simulink model "Modelo_asynchronous_machine_with_inverter"  (R2023b)
settings: Solver=ode45  StartTime=0.0  StopTime=0.5  MaxStep=1e-5  RelTol=1e-3
libraries: spsIGBTDiodeLib x6, spsVoltageMeasurementLib x3, spsAsynchronousMachineSIUnitsLib x1, simulink x1, spsDCVoltageSourceLib x1, spsThreePhaseVIMeasurementLib x1, spspowerguiLib x1
settings Model: Creator=HP  LastModifiedBy=HP

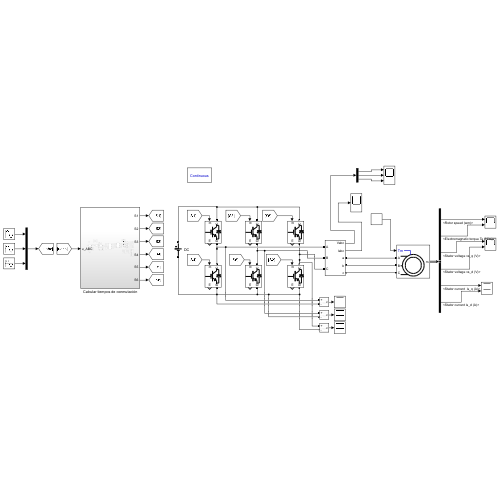
[thumbnail: Simulink's stored preview of the top-level diagram]
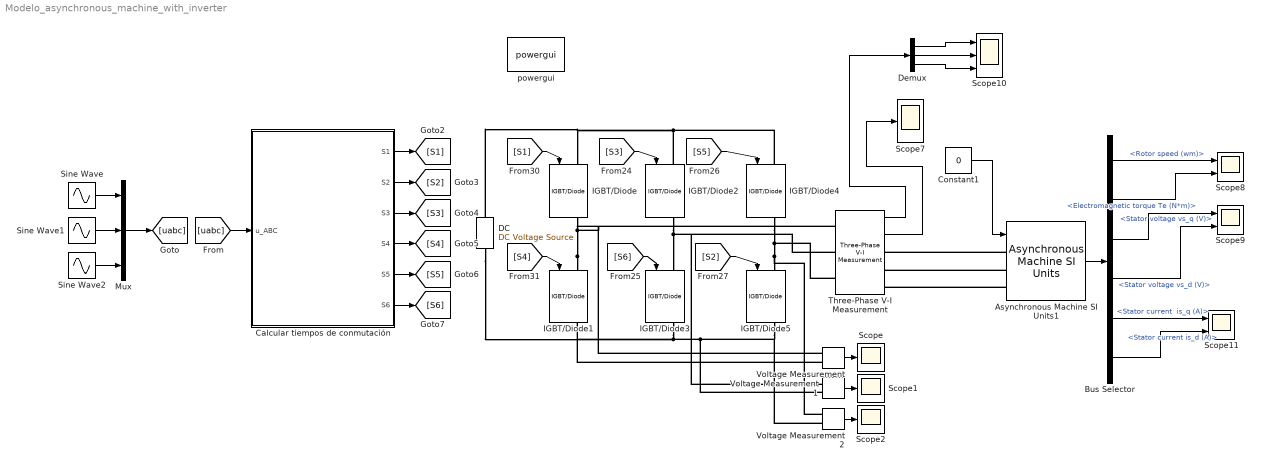
== system Modelo_asynchronous_machine_with_inverter ==
  Asynchronous Machine SI Units1 : spsAsynchronousMachineSIUnitsLib/Asynchronous Machine SI Units  RotorType=Squirrel-cage  PresetModel="01:  5 HP   460 V 60Hz 1750 RPM"  MechanicalLoad=Torque Tm  ShowDetailedParameters=on  ReferenceFrame=Rotor  Units=SI  MeasurementBus=off  NominalParameters=[3730 460 60]  VoltageRatio=1  Stator=[1.115 0.005974]  Rotor=[1.083 0.005974]  Cage1=[0.4155 0.002066]  Cage2=[0.4168 0.0003495]  Lm=0.2037  Mechanical=[0.02 0.005752 2]  PolePairs=2  InitialConditions=[1 0 0 0 0 0 0 0]  SimulateSaturation=off  Saturation=[14.03593122, 27.81365428, 53.79336849, 72.68890987, 97.98006896, 148.6815601, 215.7428561, 302.9841135, 428.7778367 ; 230, 322, 414, 460, 506, 552, 598, 644, 690]  LoadFlowParameters=1492000  TsPowergui=0  TsBlock=-1  IterativeModel=Trapezoidal non iterative  IterativeDiscreteModel=Trapezoidal non iterative  Pmec=1.492e+006
  Bus Selector : BusSelector  OutputSignals="Mechanical.Rotor speed (wm),Mechanical.Electromagnetic torque Te (N*m),Stator measurements.Stator voltage vs_q (V),Stator measurements.Stator voltage vs_d (V),Stator measurements.Stator current  is_q (A),Stator measurements.Stator current is_d (A)"
  Calcular tiempos de conmutación : Subsystem
  Constant1 : Constant  Value=0
  "DC " : spsDCVoltageSourceLib/DC Voltage Source  Amplitude=650.538  Measurements=None
  Demux : Demux  Outputs=3
  IGBT/Diode{,1..5} (6 alike) : spsIGBTDiodeLib/IGBT//Diode  Ron=1e-3  Rs=1e5  Cs=inf  Measurements=on
  Mux : Mux  Inputs=3
  Scope{,1..2,7} (4 alike) : Scope
  Scope10 : Scope  NumInputPorts=3
  Scope11 : Scope  NumInputPorts=2
  Scope8 : Scope  NumInputPorts=2
  Scope9 : Scope  NumInputPorts=2
  Sine Wave : Sin  Amplitude=375.588  Frequency=60*2*pi  SampleTime=0
  Sine Wave1 : Sin  Amplitude=375.588  Frequency=60*2*pi  Phase=2*pi/3  SampleTime=0
  Sine Wave2 : Sin  Amplitude=375.588  Frequency=60*2*pi  Phase=4*pi/3  SampleTime=0
  Three-Phase V-I Measurement : spsThreePhaseVIMeasurementLib/Three-Phase V-I Measurement  VoltageMeasurement=phase-to-phase  SetLabelV=off  LabelV=Vabc  Vpu=off  VpuLL=off  CurrentMeasurement=yes  SetLabelI=off  LabelI=Iabc  Ipu=off  Pbase=100e6  Vbase=500e3  OutputType=Complex  PhasorSimulation=off  PSBequivalent=0
  Voltage Measurement : spsVoltageMeasurementLib/Voltage Measurement  PhasorSimulation=off  OutputType=Complex  PSBequivalent=0
  Voltage Measurement1 : spsVoltageMeasurementLib/Voltage Measurement  PhasorSimulation=off  OutputType=Complex  PSBequivalent=0
  Voltage Measurement2 : spsVoltageMeasurementLib/Voltage Measurement  PhasorSimulation=off  OutputType=Complex  PSBequivalent=0
  powergui : spspowerguiLib/powergui  Priority=1  SimulationMode=Continuous  SampleTime=10e-6  frequency=60  Iterations=50  frequencyindice=0  Pbase=100e6  ErrMax=1e-4  UnitsV=kV  UnitsW=MW  buscounter=0  FunctionMessages=off  echomessages=off  EnableUseOfTLC=off  CurrentSourceSwitches=on  DisableSnubberDevices=off  DisableRonSwitches=off  DisableVfSwitches=off  DisplayEquations=off  AutomaticDiscreteSolvers=off  SolverType=Tustin/Backward Euler (TBE)  Interpol=off  ExternalGateDelay=off  methode=off  Ts=10  x0status=blocks  SPID=off  SwTol=0  HookPort=off  NonlinearTolerance=1e-4  nMaxIteration=100  ContinueOnMaxIteration=off  RestoreLinks=warning  ResistiveCurrentMeasurement=off  Frange=[0:2:500]  Ylog=off  Xlog=on  ShowGrid=off  save=off  variable=ZData  structure=ScopeData1  ZoomFFT=off  StartTime=0.0  cycles=1  DisplayStyle=1  fundamental=50  FreqAxis=off  MaxFrequency=1000  frequencyindicesteady=1  RmsSteady=1  display=off
  wires:
  Sine Wave/1 -> Mux/1
  Sine Wave1/1 -> Mux/2
  Sine Wave2/1 -> Mux/3
  Mux/1 -> [uabc]
  Demux/1 -> Scope10/1
  Demux/2 -> Scope10/2
  Constant1/1 -> Asynchronous Machine SI Units1/1
  Three-Phase V-I Measurement/2 -> Scope7/1
  Three-Phase V-I Measurement/1 -> Demux/1
  Demux/3 -> Scope10/3
  [S4] -> IGBT/Diode1/1
  [S1] -> IGBT/Diode/1
  [S3] -> IGBT/Diode2/1
  [S6] -> IGBT/Diode3/1
  [S5] -> IGBT/Diode4/1
  [S2] -> IGBT/Diode5/1
  Bus Selector/5 -> Scope11/1  "<Stator current  is_q (A)>"
  Bus Selector/2 -> Scope8/2  "<Electromagnetic torque Te (N*m)>"
  Bus Selector/4 -> Scope9/2  "<Stator voltage vs_d (V)>"
  Bus Selector/1 -> Scope8/1  "<Rotor speed (wm)>"
  Bus Selector/3 -> Scope9/1  "<Stator voltage vs_q (V)>"
  Bus Selector/6 -> Scope11/2  "<Stator current is_d (A)>"
  Asynchronous Machine SI Units1/1 -> Bus Selector/1
  Calcular tiempos de conmutación/1(S1) -> [S1]
  Calcular tiempos de conmutación/2(S2) -> [S2]
  Calcular tiempos de conmutación/3(S3) -> [S3]
  Calcular tiempos de conmutación/4(S4) -> [S4]
  Calcular tiempos de conmutación/5(S5) -> [S5]
  Calcular tiempos de conmutación/6(S6) -> [S6]
  [uabc] -> Calcular tiempos de conmutación/1(u_ABC)
  Voltage Measurement/1 -> Scope/1
  Voltage Measurement2/1 -> Scope2/1
  Voltage Measurement1/1 -> Scope1/1
  connections:
  IGBT/Diode1/LConn1 -- Voltage Measurement/LConn1 -- Three-Phase V-I Measurement/LConn1 -- IGBT/Diode/RConn1
  IGBT/Diode3/RConn1 -- Voltage Measurement2/LConn2 -- IGBT/Diode5/RConn1 -- Voltage Measurement1/LConn2 -- Voltage Measurement/LConn2 -- "DC "/LConn1 -- IGBT/Diode1/RConn1
  IGBT/Diode2/LConn1 -- "DC "/RConn1 -- IGBT/Diode/LConn1 -- IGBT/Diode4/LConn1
  IGBT/Diode2/RConn1 -- Voltage Measurement1/LConn1 -- Three-Phase V-I Measurement/LConn2 -- IGBT/Diode3/LConn1
  Three-Phase V-I Measurement/LConn3 -- IGBT/Diode4/RConn1 -- Voltage Measurement2/LConn1 -- IGBT/Diode5/LConn1
  Asynchronous Machine SI Units1/LConn1 -- Three-Phase V-I Measurement/RConn1
  Asynchronous Machine SI Units1/LConn2 -- Three-Phase V-I Measurement/RConn2
  Asynchronous Machine SI Units1/LConn3 -- Three-Phase V-I Measurement/RConn3

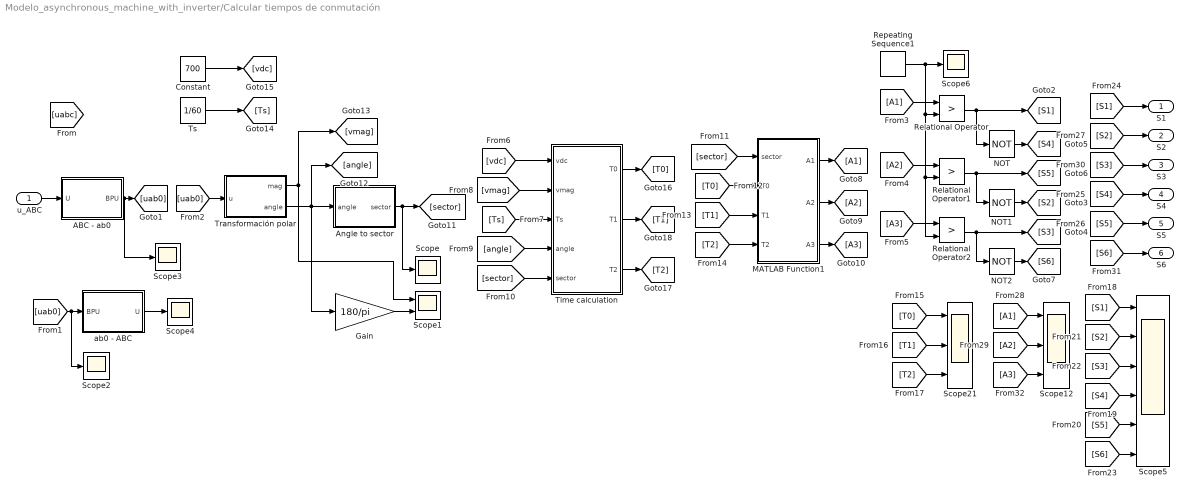
== system Modelo_asynchronous_machine_with_inverter/Calcular tiempos de conmutación ==
  u_ABC : Inport
  ABC - ab0 : MATLAB Function  TreatAsAtomicUnit=on
  Angle to sector : MATLAB Function  TreatAsAtomicUnit=on
  Constant : Constant  Value=700
  Gain : Gain  Gain=180/pi
  MATLAB Function1 : MATLAB Function  TreatAsAtomicUnit=on
  NOT : Logic  Operator=NOT  IconShape=distinctive  AllPortsSameDT=off  OutDataTypeStr=boolean
  NOT1 : Logic  Operator=NOT  IconShape=distinctive  AllPortsSameDT=off  OutDataTypeStr=boolean
  NOT2 : Logic  Operator=NOT  IconShape=distinctive  AllPortsSameDT=off  OutDataTypeStr=boolean
  Relational Operator : RelationalOperator  Operator=>  OutDataTypeStr=boolean  InputSameDT=off
  Relational Operator1 : RelationalOperator  Operator=>  OutDataTypeStr=boolean  InputSameDT=off
  Relational Operator2 : RelationalOperator  Operator=>  OutDataTypeStr=boolean  InputSameDT=off
  Repeating Sequence1 : simulink/Sources/Repeating Sequence  rep_seq_t=[0 1]*[1/5000]  rep_seq_y=[0 1/60]
  Scope{,2..4,6} (5 alike) : Scope
  Scope1 : Scope  NumInputPorts=2
  Scope12 : Scope  NumInputPorts=3
  Scope21 : Scope  NumInputPorts=3
  Scope5 : Scope  NumInputPorts=6
  Time calculation : MATLAB Function  TreatAsAtomicUnit=on
  Transformación polar : MATLAB Function  TreatAsAtomicUnit=on
  Ts : Constant  Value=1/60
  ab0 - ABC : MATLAB Function  TreatAsAtomicUnit=on
  S1 : Outport
  S2 : Outport  Port=2
  S3 : Outport  Port=3
  S4 : Outport  Port=4
  S5 : Outport  Port=5
  S6 : Outport  Port=6
  wires:
  [vmag] -> Time calculation/2(vmag)
  [sector] -> Time calculation/5(sector)
  Relational Operator2/1 -> NOT2/1, [S3]
  [Ts] -> Time calculation/3(Ts)
  NOT2/1 -> [S6]
  [S6] -> Scope5/6
  Transformación polar/1(mag) -> [vmag], Scope1/1
  [T1] -> Scope21/2
  [S3] -> Scope5/3
  Time calculation/3(T2) -> [T2]
  [T2] -> Scope21/3
  [T1] -> MATLAB Function1/3(T1)
  [uab0] -> Transformación polar/1(u)
  Time calculation/2(T1) -> [T1]
  Relational Operator1/1 -> NOT1/1, [S5]
  u_ABC/1 -> ABC - ab0/1(U)
  NOT1/1 -> [S2]
  Angle to sector/1(sector) -> [sector], Scope/1
  [S1] -> Scope5/1
  [uab0] -> Scope2/1, ab0 - ABC/1(BPU)
  [angle] -> Time calculation/4(angle)
  [S4] -> Scope5/4
  [A2] -> Relational Operator1/1
  MATLAB Function1/2(A2) -> [A2]
  NOT/1 -> [S4]
  [T2] -> MATLAB Function1/4(T2)
  Transformación polar/2(angle) -> [angle], Gain/1, Angle to sector/1(angle)
  MATLAB Function1/1(A1) -> [A1]
  Gain/1 -> Scope1/2
  Relational Operator/1 -> NOT/1, [S1]
  [A3] -> Scope12/3
  ab0 - ABC/1(U) -> Scope4/1
  ABC - ab0/1(BPU) -> Scope3/1, [uab0]
  Repeating Sequence1/1 -> Scope6/1, Relational Operator2/2, Relational Operator1/2, Relational Operator/2
  Constant/1 -> [vdc]
  [S2] -> Scope5/2
  MATLAB Function1/3(A3) -> [A3]
  [T0] -> Scope21/1
  [S5] -> Scope5/5
  [A1] -> Relational Operator/1
  [T0] -> MATLAB Function1/2(T0)
  [vdc] -> Time calculation/1(vdc)
  [sector] -> MATLAB Function1/1(sector)
  Ts/1 -> [Ts]
  [A3] -> Relational Operator2/1
  Time calculation/1(T0) -> [T0]
  [A1] -> Scope12/1
  [A2] -> Scope12/2
  [S6] -> S6/1
  [S5] -> S5/1
  [S4] -> S4/1
  [S3] -> S3/1
  [S2] -> S2/1
  [S1] -> S1/1

== matlab function Modelo_asynchronous_machine_with_inverter/Calcular tiempos de conmutación/ABC - ab0 ==
  data: U input size=[3,1]; BPU output size=[3,1]
function BPU = fcn(U)

BP = 2/3*[1,-1/2,-1/2;
          0,sqrt(3)/2,-sqrt(3)/2;
          1/2,1/2,1/2];

% Power invariant
% BP = sqrt(2/3)*[1,-1/2,-1/2;
%                 0,sqrt(3)/2,-sqrt(3)/2
%                 1/sqrt(2),1/sqrt(2),1/sqrt(2)];

BPU = BP*U;

== matlab function Modelo_asynchronous_machine_with_inverter/Calcular tiempos de conmutación/ab0 - ABC ==
  data: BPU input size=[3,1]; U output size=[3,1]
function U = fcn(BPU)

BP = 2/3*[1,-1/2,-1/2;
          0,sqrt(3)/2,-sqrt(3)/2;
          1/2,1/2,1/2];

% Power invariant
% BP = sqrt(2/3)*[1,-1/2,-1/2;
%                 0,sqrt(3)/2,-sqrt(3)/2
%                 1/sqrt(2),1/sqrt(2),1/sqrt(2)];

U = BP^-1*BPU;

== matlab function Modelo_asynchronous_machine_with_inverter/Calcular tiempos de conmutación/Transformación polar ==
  data: u input; mag output; angle output
function [mag,angle] = fcn(u)

u_alpha = u(1);
u_beta = u(2);
%u_zeta = u(3);

mag = sqrt(u_alpha^2+u_beta^2);

angle = atan2(u_beta,u_alpha);

== matlab function Modelo_asynchronous_machine_with_inverter/Calcular tiempos de conmutación/Angle to sector ==
  data: angle input; sector output
function sector = fcn(angle)

angle = angle*180/pi;

if angle >= 0 && angle <= 60
    sector = 1;
elseif angle > 60 && angle <= 120
    sector = 2;
elseif angle > 120 && angle <= 180
    sector = 3;
elseif angle > -180 && angle <= -120
    sector = 4;
elseif angle > -120 && angle <= -60
    sector = 5;
elseif angle > -60 && angle <= 0
    sector = 6;
else
    sector = -1;
end

== matlab function Modelo_asynchronous_machine_with_inverter/Calcular tiempos de conmutación/Time calculation ==
  data: vdc input; vmag input; T0 output; Ts input; angle input; sector input; T1 output; T2 output
function [T0,T1,T2] = fcn(vdc,vmag,Ts,angle,sector)

a = sqrt(3)*vmag/vdc*Ts;

T1 = a*sin(sector*pi/3 - angle);
T2 = a*sin(-(sector-1)*pi/3 + angle);

T0 = Ts - T1 - T2;

== matlab function Modelo_asynchronous_machine_with_inverter/Calcular tiempos de conmutación/MATLAB Function1 ==
  data: sector input; A1 output; T0 input; T1 input; T2 input; A2 output; A3 output
function [A1,A2,A3] = fcn(sector,T0,T1,T2)

a = T0/2;
b = T1 + T0/2;
c = T2 + T0/2;
d = T1 + T2 + T0/2;

switch sector
    case 1
        A1 = d;
        A2 = c;
        A3 = a;
    case 2
        A1 = b;
        A2 = d;
        A3 = a;
    case 3
        A1 = a;
        A2 = d;
        A3 = c;
    case 4
        A1 = a;
        A2 = b;
        A3 = d;
    case 5
        A1 = c;
        A2 = a;
        A3 = d;
    case 6
        A1 = d;
        A2 = a;
        A3 = b;
    otherwise
        A1 = -1;
        A2 = -1;
        A3 = -1;
end

%A = [A1;A2;A3];
